simulink library "Tire_Delft"  (R2025a)
settings: Solver=VariableStepAuto  StartTime=0.0  StopTime=10.0  RelTol=1e-3
libraries: sm_lib x4
Description:
  | Component of Simscape Vehicle Templates Library
  | 
  | Copyright 2018-2025 The MathWorks, Inc.
settings Model: Creator=smiller  LastModifiedBy=smiller
settings SolverCC: AlgebraicLoopSolver=TrustRegion
settings DataIOCC: ReturnWorkspaceOutputs=off
settings OptimizationCC: ReuseModelBlockBuffer=off
settings DebuggingCC: UnconnectedInputMsg=warning  UnconnectedOutputMsg=warning  UnconnectedLineMsg=warning  ArithmeticOperatorsInVariantConditions=warning
settings ModelReferenceCC: EnableRefExpFcnMdlSchedulingChecks=on
settings SFSimCC: CustomCodeUndefinedFunction=UseInterfaceOnly
settings RTWCC: GPUComputeCapability=3.5  DLArmComputeVersion=19.05

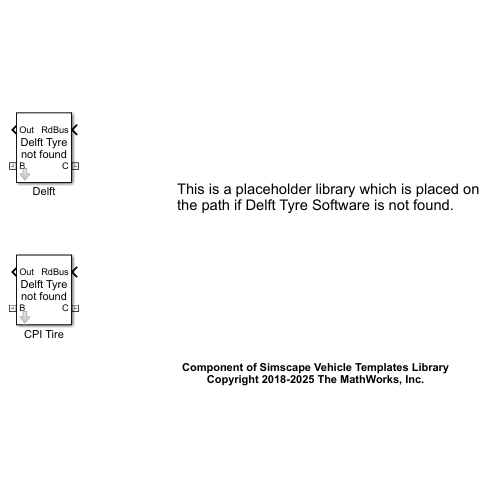
[thumbnail: Simulink's stored preview of the top-level diagram]
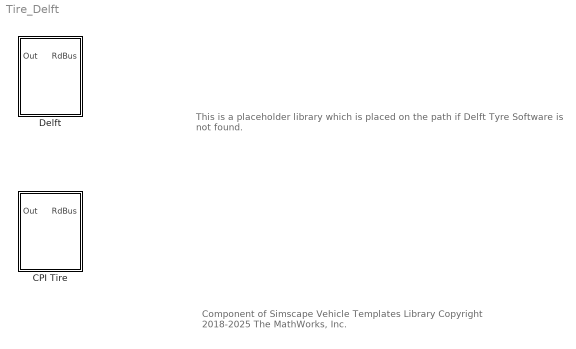
== system Tire_Delft ==
  note: This is a placeholder library which is placed on the path if Delft Tyre Software is not found.
  note: Component of Simscape Vehicle Templates Library
      | Copyright 2018-2025 The MathWorks, Inc.
  CPI Tire : Subsystem  VariantControl=CPI  mask{tireModelUnavailable=1}
      mask prompts: tireModelUnavailable "Tire Model Unavailable"
      mask help: This is a placeholder block in the event Delft Tyre software is not installed. It is here to avoid broken links and failed startup scripts only.
      mask Display: disp(sprintf('%s\n%s','Delft Tyre','not found'));
  Delft : Subsystem  VariantControl=Delft  mask{tire_side_mode=(1xxx) left, popup_leftRight=Left, tireModelUnavailable=1}
      mask prompts: tire_side_mode "Tire Side Mode (placeholder)"; popup_leftRight "Tire Side (placeholder)"; tireModelUnavailable "Tire Model Unavailable"
      mask help: This is a placeholder block in the event Delft Tyre software is not installed. It is here to avoid broken links and failed startup scripts only.
      mask TypeOptions tire_side_mode: (1xxx) left | (2xxx) right
      mask TypeOptions popup_leftRight: Left | Right
      mask DialogControl cont_tire_delft Prompt: Parameters
      mask Display: disp(sprintf('%s\n%s','Delft Tyre','not found'));

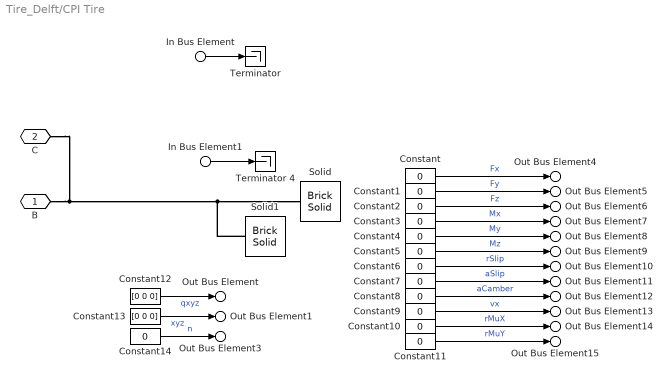
== system Tire_Delft/CPI Tire ==
  In Bus Element : Inport  PortName=RdBus  Element=gz
  In Bus Element1 : Inport  PortName=RdBus  Element=TyreScaling
  Constant{,1..11,14} (13 alike) : Constant  Value=0
  Constant12 : Constant  Value=[0 0 0]
  Constant13 : Constant  Value=[0 0 0]
  Solid : sm_lib/Body Elements/Brick Solid  BrickDimensions=[0.6 0.05 0.05]  BrickDimensionsUnits=m  ExportEntireGeometry=off  InertiaType=CalculateFromGeometry  BasedOnType=Density  Density=1000  DensityUnits=kg/m^3  Mass=1  MassUnits=kg  CenterOfMass=[0 0 0]  CenterOfMassUnits=m  MomentsOfInertia=[1 1 1]  MomentsOfInertiaUnits=kg*m^2  ProductsOfInertia=[0 0 0]  ProductsOfInertiaUnits=kg*m^2  GraphicType=FromGeometry  MarkerShape=Sphere  MarkerSize=10  GraphicVisPropType=SimpleVisualProperties  GraphicDiffuseColor=[1.0 0.0 0.0]  GraphicOpacity=1.0  GraphicSpecularColor=[0.5 0.5 0.5 1.0]  GraphicAmbientColor=[0.15 0.15 0.15 1.0]  GraphicEmissiveColor=[0.0 0.0 0.0 1.0]  GraphicShininess=75  DoExposeReferenceFrame=on  SerializedFrames=<Frames/>
  Solid1 : sm_lib/Body Elements/Brick Solid  BrickDimensions=[0.05 0.6 0.05]  BrickDimensionsUnits=m  ExportEntireGeometry=off  InertiaType=CalculateFromGeometry  BasedOnType=Density  Density=1000  DensityUnits=kg/m^3  Mass=1  MassUnits=kg  CenterOfMass=[0 0 0]  CenterOfMassUnits=m  MomentsOfInertia=[1 1 1]  MomentsOfInertiaUnits=kg*m^2  ProductsOfInertia=[0 0 0]  ProductsOfInertiaUnits=kg*m^2  GraphicType=FromGeometry  MarkerShape=Sphere  MarkerSize=10  GraphicVisPropType=SimpleVisualProperties  GraphicDiffuseColor=[1.0 0.0 0.0]  GraphicOpacity=1.0  GraphicSpecularColor=[0.5 0.5 0.5 1.0]  GraphicAmbientColor=[0.15 0.15 0.15 1.0]  GraphicEmissiveColor=[0.0 0.0 0.0 1.0]  GraphicShininess=75  DoExposeReferenceFrame=on  SerializedFrames=<Frames/>
  Terminator : Terminator
  Terminator 4 : Terminator
  B : PMIOPort  Side=Right
  C : PMIOPort  Port=2  Side=Left
  Out Bus Element : Outport  VectorParamsAs1DForOutWhenUnconnected=off  PortName=Out  Element=qxyz
  Out Bus Element1 : Outport  VectorParamsAs1DForOutWhenUnconnected=off  PortName=Out  Element=xyz
  Out Bus Element3 : Outport  VectorParamsAs1DForOutWhenUnconnected=off  PortName=Out  Element=n
  Out Bus Element4 : Outport  VectorParamsAs1DForOutWhenUnconnected=off  PortName=Out  Element=Fx
  Out Bus Element5 : Outport  VectorParamsAs1DForOutWhenUnconnected=off  PortName=Out  Element=Fy
  Out Bus Element6 : Outport  VectorParamsAs1DForOutWhenUnconnected=off  PortName=Out  Element=Fz
  Out Bus Element7 : Outport  VectorParamsAs1DForOutWhenUnconnected=off  PortName=Out  Element=Mx
  Out Bus Element8 : Outport  VectorParamsAs1DForOutWhenUnconnected=off  PortName=Out  Element=My
  Out Bus Element9 : Outport  VectorParamsAs1DForOutWhenUnconnected=off  PortName=Out  Element=Mz
  Out Bus Element10 : Outport  VectorParamsAs1DForOutWhenUnconnected=off  PortName=Out  Element=rSlip
  Out Bus Element11 : Outport  VectorParamsAs1DForOutWhenUnconnected=off  PortName=Out  Element=aSlip
  Out Bus Element12 : Outport  VectorParamsAs1DForOutWhenUnconnected=off  PortName=Out  Element=aCamber
  Out Bus Element13 : Outport  VectorParamsAs1DForOutWhenUnconnected=off  PortName=Out  Element=vx
  Out Bus Element14 : Outport  VectorParamsAs1DForOutWhenUnconnected=off  PortName=Out  Element=rMuX
  Out Bus Element15 : Outport  VectorParamsAs1DForOutWhenUnconnected=off  PortName=Out  Element=rMuY
  wires:
  Constant6/1 -> Out Bus Element10/1  "rSlip"
  Constant11/1 -> Out Bus Element15/1  "rMuY"
  In Bus Element1/1 -> Terminator 4/1
  Constant5/1 -> Out Bus Element9/1  "Mz"
  In Bus Element/1 -> Terminator/1
  Constant12/1 -> Out Bus Element/1  "qxyz"
  Constant14/1 -> Out Bus Element3/1  "n"
  Constant13/1 -> Out Bus Element1/1  "xyz"
  Constant3/1 -> Out Bus Element7/1  "Mx"
  Constant10/1 -> Out Bus Element14/1  "rMuX"
  Constant1/1 -> Out Bus Element5/1  "Fy"
  Constant8/1 -> Out Bus Element12/1  "aCamber"
  Constant7/1 -> Out Bus Element11/1  "aSlip"
  Constant4/1 -> Out Bus Element8/1  "My"
  Constant2/1 -> Out Bus Element6/1  "Fz"
  Constant9/1 -> Out Bus Element13/1  "vx"
  Constant/1 -> Out Bus Element4/1  "Fx"
  connections:
  C/RConn1 -- B/RConn1 -- Solid1/RConn1 -- Solid/RConn1

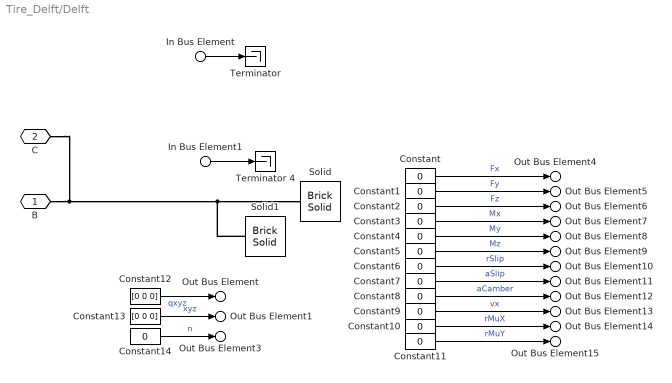
== system Tire_Delft/Delft ==
  In Bus Element : Inport  PortName=RdBus  Element=gz
  In Bus Element1 : Inport  PortName=RdBus  Element=TyreScaling
  Constant{,1..11,14} (13 alike) : Constant  Value=0
  Constant12 : Constant  Value=[0 0 0]
  Constant13 : Constant  Value=[0 0 0]
  Solid : sm_lib/Body Elements/Brick Solid  BrickDimensions=[0.6 0.05 0.05]  BrickDimensionsUnits=m  ExportEntireGeometry=off  InertiaType=CalculateFromGeometry  BasedOnType=Density  Density=1000  DensityUnits=kg/m^3  Mass=1  MassUnits=kg  CenterOfMass=[0 0 0]  CenterOfMassUnits=m  MomentsOfInertia=[1 1 1]  MomentsOfInertiaUnits=kg*m^2  ProductsOfInertia=[0 0 0]  ProductsOfInertiaUnits=kg*m^2  GraphicType=FromGeometry  MarkerShape=Sphere  MarkerSize=10  GraphicVisPropType=SimpleVisualProperties  GraphicDiffuseColor=[1.0 0.0 0.0]  GraphicOpacity=1.0  GraphicSpecularColor=[0.5 0.5 0.5 1.0]  GraphicAmbientColor=[0.15 0.15 0.15 1.0]  GraphicEmissiveColor=[0.0 0.0 0.0 1.0]  GraphicShininess=75  DoExposeReferenceFrame=on  SerializedFrames=<Frames/>
  Solid1 : sm_lib/Body Elements/Brick Solid  BrickDimensions=[0.05 0.6 0.05]  BrickDimensionsUnits=m  ExportEntireGeometry=off  InertiaType=CalculateFromGeometry  BasedOnType=Density  Density=1000  DensityUnits=kg/m^3  Mass=1  MassUnits=kg  CenterOfMass=[0 0 0]  CenterOfMassUnits=m  MomentsOfInertia=[1 1 1]  MomentsOfInertiaUnits=kg*m^2  ProductsOfInertia=[0 0 0]  ProductsOfInertiaUnits=kg*m^2  GraphicType=FromGeometry  MarkerShape=Sphere  MarkerSize=10  GraphicVisPropType=SimpleVisualProperties  GraphicDiffuseColor=[1.0 0.0 0.0]  GraphicOpacity=1.0  GraphicSpecularColor=[0.5 0.5 0.5 1.0]  GraphicAmbientColor=[0.15 0.15 0.15 1.0]  GraphicEmissiveColor=[0.0 0.0 0.0 1.0]  GraphicShininess=75  DoExposeReferenceFrame=on  SerializedFrames=<Frames/>
  Terminator : Terminator
  Terminator 4 : Terminator
  B : PMIOPort  Side=Right
  C : PMIOPort  Port=2  Side=Left
  Out Bus Element : Outport  VectorParamsAs1DForOutWhenUnconnected=off  PortName=Out  Element=qxyz
  Out Bus Element1 : Outport  VectorParamsAs1DForOutWhenUnconnected=off  PortName=Out  Element=xyz
  Out Bus Element3 : Outport  VectorParamsAs1DForOutWhenUnconnected=off  PortName=Out  Element=n
  Out Bus Element4 : Outport  VectorParamsAs1DForOutWhenUnconnected=off  PortName=Out  Element=Fx
  Out Bus Element5 : Outport  VectorParamsAs1DForOutWhenUnconnected=off  PortName=Out  Element=Fy
  Out Bus Element6 : Outport  VectorParamsAs1DForOutWhenUnconnected=off  PortName=Out  Element=Fz
  Out Bus Element7 : Outport  VectorParamsAs1DForOutWhenUnconnected=off  PortName=Out  Element=Mx
  Out Bus Element8 : Outport  VectorParamsAs1DForOutWhenUnconnected=off  PortName=Out  Element=My
  Out Bus Element9 : Outport  VectorParamsAs1DForOutWhenUnconnected=off  PortName=Out  Element=Mz
  Out Bus Element10 : Outport  VectorParamsAs1DForOutWhenUnconnected=off  PortName=Out  Element=rSlip
  Out Bus Element11 : Outport  VectorParamsAs1DForOutWhenUnconnected=off  PortName=Out  Element=aSlip
  Out Bus Element12 : Outport  VectorParamsAs1DForOutWhenUnconnected=off  PortName=Out  Element=aCamber
  Out Bus Element13 : Outport  VectorParamsAs1DForOutWhenUnconnected=off  PortName=Out  Element=vx
  Out Bus Element14 : Outport  VectorParamsAs1DForOutWhenUnconnected=off  PortName=Out  Element=rMuX
  Out Bus Element15 : Outport  VectorParamsAs1DForOutWhenUnconnected=off  PortName=Out  Element=rMuY
  wires:
  Constant1/1 -> Out Bus Element5/1  "Fy"
  Constant2/1 -> Out Bus Element6/1  "Fz"
  Constant9/1 -> Out Bus Element13/1  "vx"
  Constant7/1 -> Out Bus Element11/1  "aSlip"
  Constant10/1 -> Out Bus Element14/1  "rMuX"
  Constant/1 -> Out Bus Element4/1  "Fx"
  Constant11/1 -> Out Bus Element15/1  "rMuY"
  Constant5/1 -> Out Bus Element9/1  "Mz"
  Constant6/1 -> Out Bus Element10/1  "rSlip"
  Constant8/1 -> Out Bus Element12/1  "aCamber"
  Constant3/1 -> Out Bus Element7/1  "Mx"
  Constant4/1 -> Out Bus Element8/1  "My"
  Constant14/1 -> Out Bus Element3/1  "n"
  Constant13/1 -> Out Bus Element1/1  "xyz"
  Constant12/1 -> Out Bus Element/1  "qxyz"
  In Bus Element/1 -> Terminator/1
  In Bus Element1/1 -> Terminator 4/1
  connections:
  B/RConn1 -- Solid1/RConn1 -- Solid/RConn1 -- C/RConn1
